simulink subsystem "dc_motor_transfer_function_model"  (R2026a)
settings: Solver=VariableStepAuto
settings Model: Creator=10120  LastModifiedBy=10120

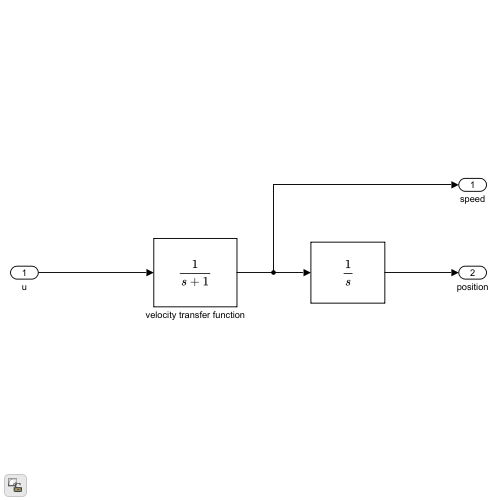
[thumbnail: Simulink's stored preview of the top-level diagram]
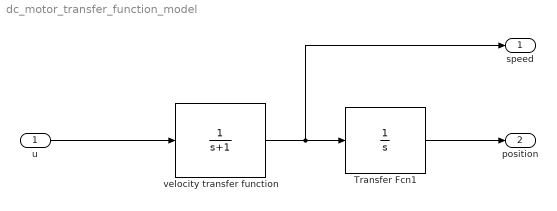
== system dc_motor_transfer_function_model ==
  u : Inport
  Transfer Fcn1 : TransferFcn  Denominator=[1 0]
  velocity transfer function : TransferFcn  Denominator=[1 1]
  speed : Outport
  position : Outport  Port=2
  wires:
  Transfer Fcn1/1 -> position/1
  u/1 -> velocity transfer function/1
  velocity transfer function/1 -> Transfer Fcn1/1, speed/1
